simulink model "obj_atteint_precis_2020a"  (R2020b)
settings: Solver=VariableStepAuto  StartTime=0.0  StopTime=20000  RelTol=1e-3
values from neighbouring files (symbols this model uses):
  A = [0 0 1 0 ... (first row only)    [Params.m]    (also in tests.m)
  B = [0 0;0 0;1 0;0 1]    [Params.m]    (also in tests.m)
  C = [1 0 0 0;0 1 0 0]    [Params.m]    (also in tests.m)
  D = zeros(2)    [Params.m]    (also in tests.m)
  hold_points = [ ... (first row only)    [Params.m]    (also in tests.m)
  Kc = lqr(A,B,Q,R)    [Params.m]    (also in closing.m; tests.m)
  Kf = Kf'    [Params.m]    (also in closing.m; tests.m)
undefined symbols (not defined in the file or in its folder): acc_pert, Kc_aug, mesure_error, tau, time_integ, umax
settings Model: Creator=aug19  LastModifiedBy=aug19
settings DebuggingCC: InheritedTsInSrcMsg=none

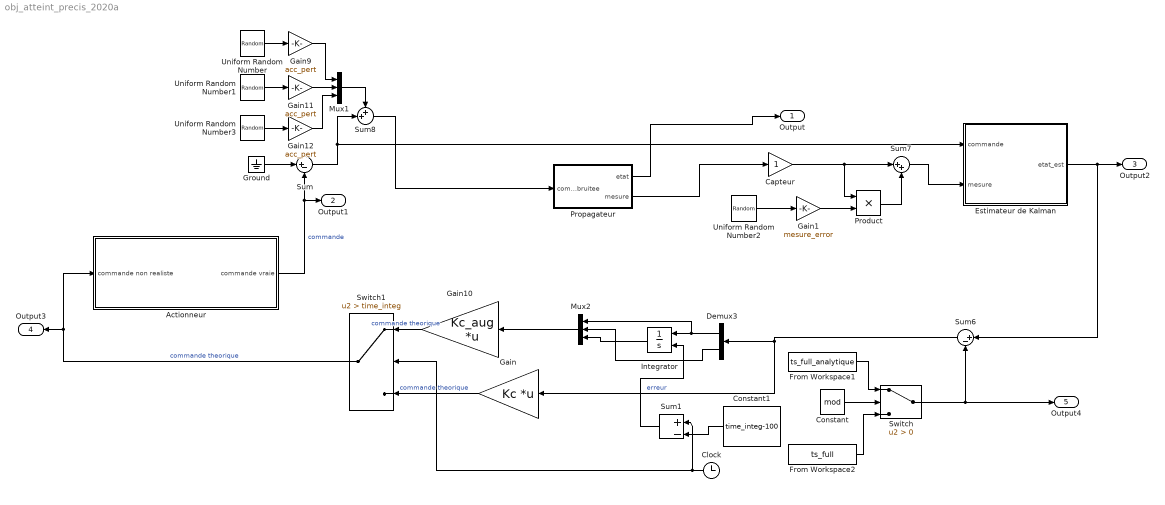
== system obj_atteint_precis_2020a ==
  Actionneur : Subsystem
  Capteur : Gain
  Clock : Clock
  Constant : Constant  Value=mod
  Constant1 : Constant  Value=time_integ-100
  Demux3 : Demux  Outputs=[3 3]
  Estimateur de Kalman : Subsystem
  From Workspace1 : FromWorkspace  VariableName=ts_full_analytique  SampleTime=-1  OutputAfterFinalValue=Holding final value
  From Workspace2 : FromWorkspace  VariableName=ts_full  SampleTime=-1  OutputAfterFinalValue=Holding final value
  Gain : Gain  Gain=Kc  Multiplication=Matrix(K*u)
  Gain1 : Gain  Gain=mesure_error
  Gain10 : Gain  Gain=Kc_aug  Multiplication=Matrix(K*u) (u vector)
  Gain11 : Gain  Gain=acc_pert
  Gain12 : Gain  Gain=acc_pert
  Gain9 : Gain  Gain=acc_pert
  Ground : Ground
  Integrator : Integrator  ExternalReset=rising
  Mux1 : Mux  Inputs=3
  Mux2 : Mux  Inputs=3
  Product : Product
  Propagateur : Subsystem
  Sum : Sum  Inputs=|+-
  Sum1 : Sum  Inputs=|+-
  Sum6 : Sum  Inputs=|+-
  Sum7 : Sum  Inputs=|++
  Sum8 : Sum  Inputs=++|
  Switch : Switch  Criteria=u2 > Threshold
  Switch1 : Switch  Criteria=u2 > Threshold  Threshold=time_integ
  Uniform Random Number : UniformRandomNumber  SampleTime=1
  Uniform Random Number1 : UniformRandomNumber  Seed=1  SampleTime=1
  Uniform Random Number2 : UniformRandomNumber  Seed=3  SampleTime=1
  Uniform Random Number3 : UniformRandomNumber  Seed=2  SampleTime=1
  Output : Outport  SignalName=etat
  Output1 : Outport  Port=2  SignalName=commande
  Output2 : Outport  Port=3  SignalName=etat_est
  Output3 : Outport  Port=4  SignalName=commande
  Output4 : Outport  Port=5  SignalName=objectif
  wires:
  Mux1/1 -> Sum8/1
  Sum8/1 -> Propagateur/1(commande bruitee)
  Gain9/1 -> Mux1/1
  Sum/1 -> Estimateur de Kalman/1(commande), Sum8/2
  Uniform Random Number3/1 -> Gain12/1
  Uniform Random Number2/1 -> Gain1/1
  Uniform Random Number/1 -> Gain9/1
  Constant/1 -> Switch/2
  From Workspace1/1 -> Switch/1
  Switch/1 -> Output4/1, Sum6/2
  Gain12/1 -> Mux1/3
  Gain11/1 -> Mux1/2
  Uniform Random Number1/1 -> Gain11/1
  From Workspace2/1 -> Switch/3
  Product/1 -> Sum7/2
  Mux2/1 -> Gain10/1
  Integrator/1 -> Mux2/3
  Switch1/1 -> Actionneur/1(commande non realiste), Output3/1  "commande theorique"
  Sum6/1 -> Demux3/1, Gain/1  "erreur"
  Demux3/1 -> Mux2/1, Integrator/1
  Demux3/2 -> Mux2/2
  Capteur/1 -> Product/1, Sum7/1
  Actionneur/1(commande vraie) -> Sum/2, Output1/1  "commande"
  Propagateur/1(etat) -> Output/1
  Propagateur/2(mesure) -> Capteur/1
  Estimateur de Kalman/1(etat_est) -> Output2/1, Sum6/1
  Sum7/1 -> Estimateur de Kalman/2(mesure)
  Ground/1 -> Sum/1
  Gain10/1 -> Switch1/1  "commande theorique"
  Gain/1 -> Switch1/3  "commande theorique"
  Clock/1 -> Sum1/1, Switch1/2
  Sum1/1 -> Integrator/2
  Constant1/1 -> Sum1/2
  Gain1/1 -> Product/2

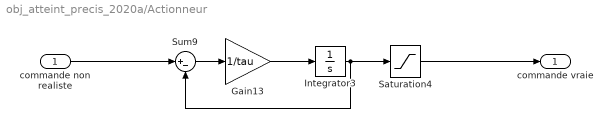
== system obj_atteint_precis_2020a/Actionneur ==
  commande non realiste : Inport
  Gain13 : Gain  Gain=1/tau
  Integrator3 : Integrator  InitialCondition=[0,0,0]
  Saturation4 : Saturate  UpperLimit=umax  LowerLimit=-umax
  Sum9 : Sum  Inputs=|+-
  commande vraie : Outport
  wires:
  Gain13/1 -> Integrator3/1
  Integrator3/1 -> Saturation4/1, Sum9/2
  commande non realiste/1 -> Sum9/1
  Saturation4/1 -> commande vraie/1
  Sum9/1 -> Gain13/1

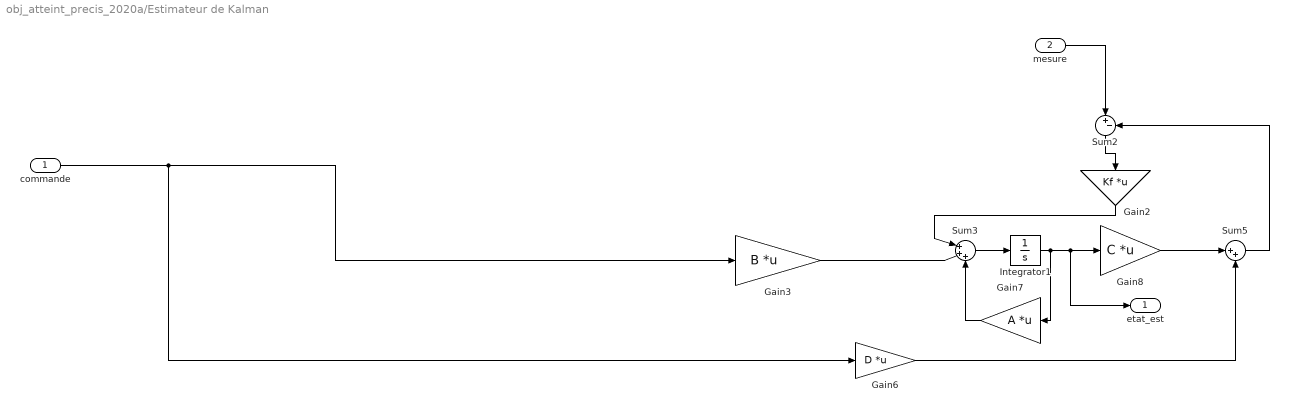
== system obj_atteint_precis_2020a/Estimateur de Kalman ==
  commande : Inport
  mesure : Inport  Port=2
  Gain2 : Gain  Gain=Kf  Multiplication=Matrix(K*u) (u vector)
  Gain3 : Gain  Gain=B  Multiplication=Matrix(K*u) (u vector)
  Gain6 : Gain  Gain=D  Multiplication=Matrix(K*u) (u vector)
  Gain7 : Gain  Gain=A  Multiplication=Matrix(K*u) (u vector)
  Gain8 : Gain  Gain=C  Multiplication=Matrix(K*u) (u vector)
  Integrator1 : Integrator  InitialCondition=hold_points(1,:)
  Sum2 : Sum  Inputs=|+-
  Sum3 : Sum  Inputs=|+++
  Sum5 : Sum  Inputs=|++
  etat_est : Outport
  wires:
  Gain6/1 -> Sum5/2
  Gain7/1 -> Sum3/3
  Sum2/1 -> Gain2/1
  Gain3/1 -> Sum3/2
  Gain8/1 -> Sum5/1
  Gain2/1 -> Sum3/1
  Integrator1/1 -> etat_est/1, Gain8/1, Gain7/1
  Sum3/1 -> Integrator1/1
  Sum5/1 -> Sum2/2
  commande/1 -> Gain6/1, Gain3/1
  mesure/1 -> Sum2/1

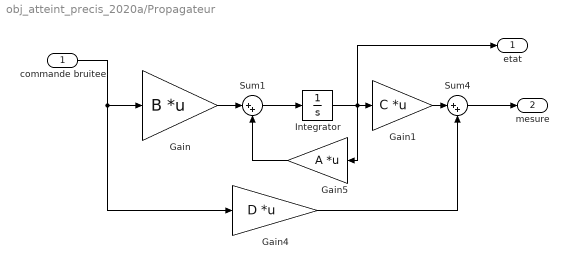
== system obj_atteint_precis_2020a/Propagateur ==
  commande bruitee : Inport
  Gain : Gain  Gain=B  Multiplication=Matrix(K*u) (u vector)
  Gain1 : Gain  Gain=C  Multiplication=Matrix(K*u) (u vector)
  Gain4 : Gain  Gain=D  Multiplication=Matrix(K*u) (u vector)
  Gain5 : Gain  Gain=A  Multiplication=Matrix(K*u) (u vector)
  Integrator : Integrator  InitialCondition=hold_points(1,:)
  Sum1 : Sum  Inputs=|++
  Sum4 : Sum  Inputs=|++
  etat : Outport
  mesure : Outport  Port=2
  wires:
  Gain/1 -> Sum1/1
  commande bruitee/1 -> Gain4/1, Gain/1
  Integrator/1 -> etat/1, Gain5/1, Gain1/1
  Gain5/1 -> Sum1/2
  Gain4/1 -> Sum4/2
  Gain1/1 -> Sum4/1
  Sum1/1 -> Integrator/1
  Sum4/1 -> mesure/1
